simulink model "integral_controller_with_obsever"  (R2016a)
settings: Solver=VariableStepAuto  StartTime=0.0  StopTime=0.2  RelTol=1e-5
undefined symbols (not defined in the file or in its folder): A, B, C, K, Ko
settings Model: Creator=manuel  LastModifiedBy=manuel

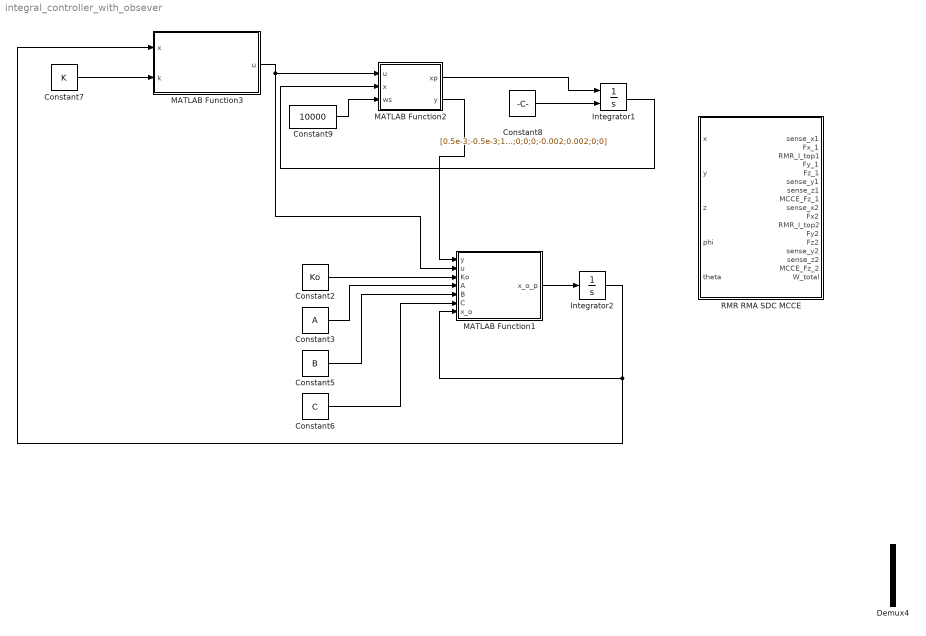
== system integral_controller_with_obsever ==
  Constant2 : Constant  Value=Ko  VectorParams1D=off
  Constant3 : Constant  Value=A  VectorParams1D=off
  Constant5 : Constant  Value=B  VectorParams1D=off
  Constant6 : Constant  Value=C  VectorParams1D=off
  Constant7 : Constant  Value=K  VectorParams1D=off
  Constant8 : Constant  Value=[0.5e-3;-0.5e-3;1e-3;0;0;0;-0.002;0.002;0;0]
  Constant9 : Constant  Value=10000  VectorParams1D=off
  Demux4 : Demux  Outputs=3
  Integrator1 : Integrator  InitialConditionSource=external
  Integrator2 : Integrator  InitialCondition=[0;0;0;0;0;0;0;0;0;0]
  MATLAB Function1 : MATLAB Function  TreatAsAtomicUnit=on
  MATLAB Function2 : MATLAB Function  TreatAsAtomicUnit=on
  MATLAB Function3 : MATLAB Function  TreatAsAtomicUnit=on
  RMR RMA SDC MCCE : Subsystem
  wires:
  Constant8/1 -> Integrator1/2
  Integrator1/1 -> MATLAB Function2/2(x)
  Constant7/1 -> MATLAB Function3/2(k)
  MATLAB Function2/1(xp) -> Integrator1/1
  MATLAB Function2/2(y) -> MATLAB Function1/1(y)
  MATLAB Function1/1(x_o_p) -> Integrator2/1
  Constant2/1 -> MATLAB Function1/3(Ko)
  Constant3/1 -> MATLAB Function1/4(A)
  Constant5/1 -> MATLAB Function1/5(B)
  Constant6/1 -> MATLAB Function1/6(C)
  Integrator2/1 -> MATLAB Function3/1(x), MATLAB Function1/7(x_o)
  MATLAB Function3/1(u) -> MATLAB Function1/2(u), MATLAB Function2/1(u)
  Constant9/1 -> MATLAB Function2/3(ws)

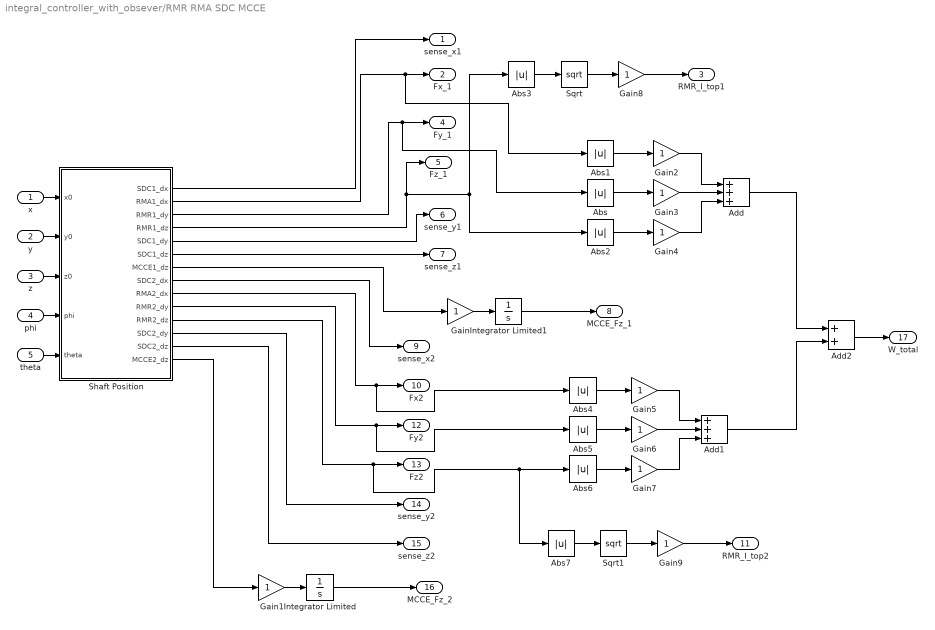
== system integral_controller_with_obsever/RMR RMA SDC MCCE ==
  x : Inport
  y : Inport  Port=2
  z : Inport  Port=3
  phi : Inport  Port=4
  theta : Inport  Port=5
  Abs{,1..7} (8 alike) : Abs
  Add : Sum  Inputs=+++
  Add1 : Sum  Inputs=+++
  Add2 : Sum
  Gain{,1..9} (10 alike) : Gain
  Integrator Limited : Integrator  LimitOutput=on  UpperSaturationLimit=1  LowerSaturationLimit=0
  Integrator Limited1 : Integrator  LimitOutput=on  UpperSaturationLimit=1  LowerSaturationLimit=0
  Shaft Position : MATLAB Function  TreatAsAtomicUnit=on
  Sqrt : Sqrt  SaturateOnIntegerOverflow=on
  Sqrt1 : Sqrt  SaturateOnIntegerOverflow=on
  sense_x1 : Outport
  Fx_1 : Outport  Port=2
  RMR_I_top1 : Outport  Port=3
  Fy_1 : Outport  Port=4
  Fz_1 : Outport  Port=5
  sense_y1 : Outport  Port=6
  sense_z1 : Outport  Port=7
  MCCE_Fz_1 : Outport  Port=8
  sense_x2 : Outport  Port=9
  Fx2 : Outport  Port=10
  RMR_I_top2 : Outport  Port=11
  Fy2 : Outport  Port=12
  Fz2 : Outport  Port=13
  sense_y2 : Outport  Port=14
  sense_z2 : Outport  Port=15
  MCCE_Fz_2 : Outport  Port=16
  W_total : Outport  Port=17
  wires:
  y/1 -> Shaft Position/2(y0)
  x/1 -> Shaft Position/1(x0)
  z/1 -> Shaft Position/3(z0)
  phi/1 -> Shaft Position/4(phi)
  theta/1 -> Shaft Position/5(theta)
  Add/1 -> Add2/1
  Shaft Position/1(SDC1_dx) -> sense_x1/1
  Shaft Position/3(RMR1_dy) -> Fy_1/1, Abs/1
  Shaft Position/4(RMR1_dz) -> Fz_1/1, Abs2/1, Abs3/1
  Shaft Position/5(SDC1_dy) -> sense_y1/1
  Shaft Position/6(SDC1_dz) -> sense_z1/1
  Gain/1 -> Integrator Limited1/1
  Shaft Position/7(MCCE1_dz) -> Gain/1
  Integrator Limited1/1 -> MCCE_Fz_1/1
  Shaft Position/12(SDC2_dy) -> sense_y2/1
  Shaft Position/13(SDC2_dz) -> sense_z2/1
  Shaft Position/14(MCCE2_dz) -> Gain1/1
  Gain3/1 -> Add/2
  Gain2/1 -> Add/1
  Gain4/1 -> Add/3
  Shaft Position/2(RMA1_dx) -> Abs1/1, Fx_1/1
  Add1/1 -> Add2/2
  Shaft Position/9(RMA2_dx) -> Abs4/1, Fx2/1
  Shaft Position/10(RMR2_dy) -> Abs5/1, Fy2/1
  Gain6/1 -> Add1/2
  Gain5/1 -> Add1/1
  Gain7/1 -> Add1/3
  Shaft Position/8(SDC2_dx) -> sense_x2/1
  Shaft Position/11(RMR2_dz) -> Abs7/1, Abs6/1, Fz2/1
  Add2/1 -> W_total/1
  Sqrt/1 -> Gain8/1
  Gain8/1 -> RMR_I_top1/1
  Abs1/1 -> Gain2/1
  Abs/1 -> Gain3/1
  Abs2/1 -> Gain4/1
  Abs3/1 -> Sqrt/1
  Abs4/1 -> Gain5/1
  Abs5/1 -> Gain6/1
  Abs6/1 -> Gain7/1
  Sqrt1/1 -> Gain9/1
  Gain9/1 -> RMR_I_top2/1
  Abs7/1 -> Sqrt1/1
  Gain1/1 -> Integrator Limited/1
  Integrator Limited/1 -> MCCE_Fz_2/1

== matlab function integral_controller_with_obsever/MATLAB Function1 ==
  data: y input; u input; x_o_p output; Ko input; A input; B input; C input; x_o input
function x_o_p = state_obsever(y,u,Ko,A,B,C,x_o)
%#codegen
x_o_p = A*x_o + B*u + Ko*(y-C*x_o);

== matlab function integral_controller_with_obsever/MATLAB Function2 ==
  data: u input; x input; xp output; y output; ws input
function [xp,y] = fcn(u,x,ws)

Fd_x = 0;
Fd_y = 0;
Fd_z = 0;
Md_y = 0;
Md_z = 0;
[xp,y] = hmb_non_linear_model(x,u,ws,Fd_x,Fd_y,Fd_z,Md_y,Md_z);

end

== matlab function integral_controller_with_obsever/MATLAB Function3 ==
  data: x input; k input; u output
function u = feedback_controller(x,k)
%#codegen
u = -k*x;

== matlab function integral_controller_with_obsever/RMR RMA SDC MCCE/Shaft Position ==
  data: x0 input; SDC1_dx output; y0 input; z0 input; phi input; theta input; RMA1_dx output; RMR1_dy output; RMR1_dz output; SDC1_dy output; SDC1_dz output; MCCE1_dz output; SDC2_dx output; RMA2_dx output; RMR2_dy output; RMR2_dz output; SDC2_dy output; SDC2_dz output; MCCE2_dz output
function [SDC1_dx, RMA1_dx, RMR1_dy, RMR1_dz, SDC1_dy, SDC1_dz, MCCE1_dz, SDC2_dx, RMA2_dx, RMR2_dy, RMR2_dz, SDC2_dy, SDC2_dz, MCCE2_dz] = fcn(x0,y0,z0,phi,theta)
%#codegen
SDC1_dx = 0;
RMA1_dx = 0;
RMR1_dy = 0;
RMR1_dz = 0;
SDC1_dy = 0;
SDC1_dz = 0;
MCCE1_dz = 0;

SDC2_dx = 0;
RMA2_dx = 0;
RMR2_dy = 0;
RMR2_dz = 0;
SDC2_dy = 0;
SDC2_dz = 0;
MCCE2_dz = 0;
